simulink model "prob_6"  (R2015a)
settings: Solver=ode45  StartTime=0.0  StopTime=1  RelTol=1e-3
settings Model: Creator=Anu  LastModifiedBy=Anu

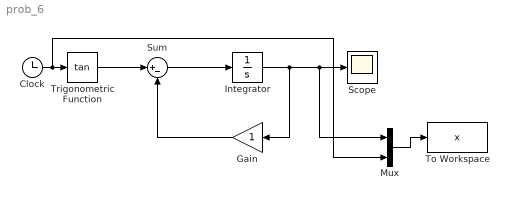
== system prob_6 ==
  Clock : Clock
  Gain : Gain
  Integrator : Integrator
  Mux : Mux  Inputs=2
  Scope : Scope
  Sum : Sum  Inputs=|+-
  To Workspace : ToWorkspace  VariableName=x  SampleTime=-1
  Trigonometric Function : Trigonometry  Operator=tan
  wires:
  Trigonometric Function/1 -> Sum/1
  Gain/1 -> Sum/2
  Sum/1 -> Integrator/1
  Integrator/1 -> Gain/1, Mux/1, Scope/1
  Clock/1 -> Mux/2, Trigonometric Function/1
  Mux/1 -> To Workspace/1
